simulink model "c09f12_01_avn"  (R2012b)
settings: Solver=ode45  StartTime=0.0  StopTime="(2^(7+2))  * (2^8)"  RelTol=1e-3
undefined symbols (not defined in the file): Down, pfb_coeff_gen_calc, Up, xlipgetpartsetting
libraries: xbsIndex_r4 x7041, casper_library_misc x193, xps_library x58, casper_library_delays x50, simulink x16, dspsigops x12, casper_library_flow_control x5, xbsReplacements_r4 x4, casper_library_ffts_twiddle x2, casper_library_multipliers x2, casper_library_reorder x1
(part 3 of 77)

== system c09f12_01_avn/calc_adc_sum_sq ==
  In1 : Inport
  In2 : Inport  Port=2
  In3 : Inport  Port=3
  In4 : Inport  Port=4
  Accumulator : xbsIndex_r4/Accumulator  operation=Add  n_bits=32  overflow=Wrap  scale=1  rst=on  infoeditControl=reset for floating point data type must be asserted for a minimum of 2 cycles  hasbypass=off  en=off  latency=0  dbl_ovrd=off  msb_inp=100  msb=100  lsb=-100  use_behavioral_HDL=off  implementation=DSP48  block_type=accum
      settings: xl_area=[0, 0, 0, 0, 0, 0, 0]  block_version=10.1.3
  Convert1 : xbsIndex_r4/Convert  gui_display_data_type=Fixed-point  arith_type=Unsigned  n_bits=32  bin_pt=0  float_type=Single  exp_bits=8  fraction_bits=24  quantization=Truncate  overflow=Wrap  en=off  latency=0  dbl_ovrd=off  pipeline=off  block_type=convert
      settings: block_version=11.4
  Counter : xbsIndex_r4/Counter  cnt_type=Free Running  cnt_to=Inf  operation=Up  start_count=0  cnt_by_val=1  arith_type=Unsigned  n_bits=2  bin_pt=0  load_pin=off  rst=off  en=off  explicit_period=off  period=1  dbl_ovrd=off  use_behavioral_HDL=off  implementation=Fabric  use_rpm=on  block_type=counter
      settings: xl_area=[0, 0, 0, 0, 0, 0, 0]
  Counter1 : xbsIndex_r4/Counter  cnt_type=Free Running  cnt_to=Inf  operation=Up  start_count=0  cnt_by_val=1  arith_type=Unsigned  n_bits=16  bin_pt=0  load_pin=off  rst=off  en=off  explicit_period=on  period=1  dbl_ovrd=off  use_behavioral_HDL=off  implementation=DSP48  use_rpm=on  block_type=counter
      settings: xl_area=[0, 0, 0, 0, 0, 0, 0]
  Delay : xbsIndex_r4/Delay  rst=off  infoeditControl=Selection of Reset will increase slice count due to use of real FFs and instead of SRLs  en=off  latency=1  dbl_ovrd=off  reg_retiming=on  block_type=delay
      settings: block_version=11.4
  Delay1 : xbsIndex_r4/Delay  rst=off  infoeditControl=Selection of Reset will increase slice count due to use of real FFs and instead of SRLs  en=off  latency=1  dbl_ovrd=off  reg_retiming=on  block_type=delay
      settings: block_version=11.4
  Mult : xbsIndex_r4/Mult  precision=Full  arith_type="Signed  (2's comp)"  n_bits=8  bin_pt=2  quantization=Truncate  overflow=Wrap  en=off  latency=2  dbl_ovrd=off  use_behavioral_HDL=on  opt=Speed  use_embedded=on  optimum_pipeline=off  pipeline=on  use_rpm=on  placement_style=Rectangular shape  block_type=mult
      settings: xl_area=[0, 0, 0, 0, 0, 0, 0]  block_version=10.1.3
  Mux : xbsIndex_r4/Mux  inputs=4  en=off  latency=1  precision=Full  arith_type="Signed  (2's comp)"  n_bits=8  bin_pt=2  quantization=Truncate  overflow=Wrap  dbl_ovrd=off  block_type=mux
      settings: xl_area=[0, 0, 0, 0, 0, 0, 0]
  Register : xbsIndex_r4/Register  init=0  rst=off  en=on  dbl_ovrd=off  block_type=register
      settings: xl_area=[0, 0, 0, 0, 0, 0, 0]
  Slice : xbsIndex_r4/Slice  nbits=1  boolean_output=on  mode=Upper Bit Location + Width  bit1=0  base1=MSB of Input  bit0=0  base0=LSB of Input  dbl_ovrd=off  block_type=slice
      settings: block_version=10.1.3
  edge_detect1 : Subsystem  AncestorBlock=casper_library_misc/edge_detect  mask(edge_detect){edge=Falling, polarity=Active High, x_in=[0 0.08 0.08 0.16 0.16 0.24 0.24 0.32 0.32 0.4], y_in=[1  1 -1 -1 -1 -1 -1 -1 -1 -1], x_out=[0.6 0.68 0.68 0.76 0.76 0.84 0.84 0.92 0.92 1], y_out=[-1 -1  1  1 -1 -1 -1 -1 -1 -1]}
      mask prompts: edge "Edge Type"; polarity "Output Polarity"; x_in "Input X Positions"; y_in "Input Y Positions"; x_out "Output X Positions"; y_out "Output Y Positions"
      mask help: Output is active for one-cycle after each edge of the specified type (i.e. rising, falling or both).
      mask init: same as c09f12_01_avn/edge_detect2
      settings: AttributesFormatString=|
      | falling edges
      | active high
      mask Help: Output is active for one-cycle after each edge of the specified type (i.e. rising, falling, or both).  Latency is zero.
      mask TypeOptions edge: Rising | Falling | Both
      mask TypeOptions polarity: Active High | Active Low
      mask Display:
      | plot(x_in_num,0.5+y_in_num*0.2);
      | plot(x_out_num,0.5+y_out_num*0.2);
  sum_sq : Outport
  wires:
  Mult/1 -> Delay/1
  Accumulator/1 -> Register/1
  Register/1 -> Convert1/1
  Mux/1 -> Mult/1, Mult/2
  Counter/1 -> Mux/1
  Counter1/1 -> Slice/1
  Slice/1 -> edge_detect1/1(in)
  edge_detect1/1(out) -> Delay1/1
  In1/1 -> Mux/2
  In3/1 -> Mux/3
  In2/1 -> Mux/4
  In4/1 -> Mux/5
  Convert1/1 -> sum_sq/1
  Delay/1 -> Accumulator/1
  Delay1/1 -> Accumulator/2, Register/2

== system c09f12_01_avn/calc_adc_sum_sq1 ==
  In1 : Inport
  In2 : Inport  Port=2
  In3 : Inport  Port=3
  In4 : Inport  Port=4
  Accumulator : xbsIndex_r4/Accumulator  operation=Add  n_bits=32  overflow=Wrap  scale=1  rst=on  infoeditControl=reset for floating point data type must be asserted for a minimum of 2 cycles  hasbypass=off  en=off  latency=0  dbl_ovrd=off  msb_inp=100  msb=100  lsb=-100  use_behavioral_HDL=off  implementation=DSP48  block_type=accum
      settings: xl_area=[0, 0, 0, 0, 0, 0, 0]  block_version=10.1.3
  Convert1 : xbsIndex_r4/Convert  gui_display_data_type=Fixed-point  arith_type=Unsigned  n_bits=32  bin_pt=0  float_type=Single  exp_bits=8  fraction_bits=24  quantization=Truncate  overflow=Wrap  en=off  latency=0  dbl_ovrd=off  pipeline=off  block_type=convert
      settings: block_version=11.4
  Counter : xbsIndex_r4/Counter  cnt_type=Free Running  cnt_to=Inf  operation=Up  start_count=0  cnt_by_val=1  arith_type=Unsigned  n_bits=2  bin_pt=0  load_pin=off  rst=off  en=off  explicit_period=off  period=1  dbl_ovrd=off  use_behavioral_HDL=off  implementation=Fabric  use_rpm=on  block_type=counter
      settings: xl_area=[0, 0, 0, 0, 0, 0, 0]
  Counter1 : xbsIndex_r4/Counter  cnt_type=Free Running  cnt_to=Inf  operation=Up  start_count=0  cnt_by_val=1  arith_type=Unsigned  n_bits=16  bin_pt=0  load_pin=off  rst=off  en=off  explicit_period=on  period=1  dbl_ovrd=off  use_behavioral_HDL=off  implementation=DSP48  use_rpm=on  block_type=counter
      settings: xl_area=[0, 0, 0, 0, 0, 0, 0]
  Delay : xbsIndex_r4/Delay  rst=off  infoeditControl=Selection of Reset will increase slice count due to use of real FFs and instead of SRLs  en=off  latency=1  dbl_ovrd=off  reg_retiming=on  block_type=delay
      settings: block_version=11.4
  Delay1 : xbsIndex_r4/Delay  rst=off  infoeditControl=Selection of Reset will increase slice count due to use of real FFs and instead of SRLs  en=off  latency=1  dbl_ovrd=off  reg_retiming=on  block_type=delay
      settings: block_version=11.4
  Mult : xbsIndex_r4/Mult  precision=Full  arith_type="Signed  (2's comp)"  n_bits=8  bin_pt=2  quantization=Truncate  overflow=Wrap  en=off  latency=2  dbl_ovrd=off  use_behavioral_HDL=on  opt=Speed  use_embedded=on  optimum_pipeline=off  pipeline=on  use_rpm=on  placement_style=Rectangular shape  block_type=mult
      settings: xl_area=[0, 0, 0, 0, 0, 0, 0]  block_version=10.1.3
  Mux : xbsIndex_r4/Mux  inputs=4  en=off  latency=1  precision=Full  arith_type="Signed  (2's comp)"  n_bits=8  bin_pt=2  quantization=Truncate  overflow=Wrap  dbl_ovrd=off  block_type=mux
      settings: xl_area=[0, 0, 0, 0, 0, 0, 0]
  Register : xbsIndex_r4/Register  init=0  rst=off  en=on  dbl_ovrd=off  block_type=register
      settings: xl_area=[0, 0, 0, 0, 0, 0, 0]
  Slice : xbsIndex_r4/Slice  nbits=1  boolean_output=on  mode=Upper Bit Location + Width  bit1=0  base1=MSB of Input  bit0=0  base0=LSB of Input  dbl_ovrd=off  block_type=slice
      settings: block_version=10.1.3
  edge_detect1 : Subsystem  AncestorBlock=casper_library_misc/edge_detect  mask(edge_detect){edge=Falling, polarity=Active High, x_in=[0 0.08 0.08 0.16 0.16 0.24 0.24 0.32 0.32 0.4], y_in=[1  1 -1 -1 -1 -1 -1 -1 -1 -1], x_out=[0.6 0.68 0.68 0.76 0.76 0.84 0.84 0.92 0.92 1], y_out=[-1 -1  1  1 -1 -1 -1 -1 -1 -1]}
      mask prompts: edge "Edge Type"; polarity "Output Polarity"; x_in "Input X Positions"; y_in "Input Y Positions"; x_out "Output X Positions"; y_out "Output Y Positions"
      mask help: Output is active for one-cycle after each edge of the specified type (i.e. rising, falling or both).
      mask init: same as c09f12_01_avn/edge_detect2
      settings: AttributesFormatString=|
      | falling edges
      | active high
      mask Help: Output is active for one-cycle after each edge of the specified type (i.e. rising, falling, or both).  Latency is zero.
      mask TypeOptions edge: Rising | Falling | Both
      mask TypeOptions polarity: Active High | Active Low
      mask Display:
      | plot(x_in_num,0.5+y_in_num*0.2);
      | plot(x_out_num,0.5+y_out_num*0.2);
  sum_sq : Outport
  wires:
  Delay1/1 -> Register/2, Accumulator/2
  Delay/1 -> Accumulator/1
  Convert1/1 -> sum_sq/1
  In4/1 -> Mux/5
  In2/1 -> Mux/4
  In3/1 -> Mux/3
  In1/1 -> Mux/2
  edge_detect1/1(out) -> Delay1/1
  Slice/1 -> edge_detect1/1(in)
  Counter1/1 -> Slice/1
  Counter/1 -> Mux/1
  Mux/1 -> Mult/2, Mult/1
  Register/1 -> Convert1/1
  Accumulator/1 -> Register/1
  Mult/1 -> Delay/1

== system c09f12_01_avn/cd_local_time ==
  note: A reset pulse resets
      | the clock which starts
      | counting at the next sync
  reset : Inport
  sync : Inport  Port=2
  Delay : xbsIndex_r4/Delay  rst=off  infoeditControl=Selection of Reset will increase slice count due to use of real FFs and instead of SRLs  en=off  latency=1  dbl_ovrd=off  reg_retiming=on  block_type=delay
  Register : xbsIndex_r4/Register  init=0  rst=on  en=on  dbl_ovrd=off  block_type=register
  clock : xbsIndex_r4/Counter  cnt_type=Free Running  cnt_to=Inf  operation=Up  start_count=0  cnt_by_val=1  arith_type=Unsigned  n_bits=64  bin_pt=0  load_pin=off  rst=on  en=on  explicit_period=on  period=1  dbl_ovrd=off  use_behavioral_HDL=off  implementation=Fabric  use_rpm=on  block_type=counter
  edge_detect1 : casper_library_misc/edge_detect  edge=Rising  polarity=Active High  x_in=[0 0.08 0.08 0.16 0.16 0.24 0.24 0.32 0.32 0.4]  y_in="[-1 -1  1  1  1  1  1  1  1  1]"  x_out=[0.6 0.68 0.68 0.76 0.76 0.84 0.84 0.92 0.92 1]  y_out="[-1 -1  1  1 -1 -1 -1 -1 -1 -1]"
  time : Outport
  wires:
  clock/1 -> time/1
  sync/1 -> Register/1, Register/3
  reset/1 -> Register/2, edge_detect1/1
  Register/1 -> clock/2
  edge_detect1/1 -> Delay/1
  Delay/1 -> clock/1

== system c09f12_01_avn/coarse ==
  sync : Inport
  data0 : Inport  Port=2
  data1 : Inport  Port=3
  fft_shift : Inport  Port=4
  channel_select : Inport  Port=5
  debug_polsel : Inport  Port=6
  debug_chansel : Inport  Port=7
  debug_chan : Inport  Port=8
  1st_shift : Subsystem  mask{shift=fftShift, latency=0}
      mask prompts: shift "Number bits to shift right by"; latency "Shift latency"
  1st_shift1 : Subsystem  mask{shift=fftShift, latency=0}
      mask prompts: shift "Number bits to shift right by"; latency "Shift latency"
  Delay1 : xbsIndex_r4/Delay  rst=off  infoeditControl=Selection of Reset will increase slice count due to use of real FFs and instead of SRLs  en=off  latency=1  dbl_ovrd=off  reg_retiming=on  block_type=delay
      settings: block_version=11.4
  Delay2 : xbsIndex_r4/Delay  rst=off  infoeditControl=Selection of Reset will increase slice count due to use of real FFs and instead of SRLs  en=off  latency=1  dbl_ovrd=off  reg_retiming=on  block_type=delay
      settings: block_version=11.4
  Delay3 : xbsIndex_r4/Delay  rst=off  infoeditControl=Selection of Reset will increase slice count due to use of real FFs and instead of SRLs  en=off  latency=1  dbl_ovrd=off  reg_retiming=on  block_type=delay
      settings: block_version=11.4
  Mux1 : xbsIndex_r4/Mux  inputs=2  en=off  latency=1  precision=Full  arith_type=Unsigned  n_bits=16  bin_pt=14  quantization=Truncate  overflow=Wrap  dbl_ovrd=off  block_type=mux
      settings: block_version=11.4
  Mux2 : xbsIndex_r4/Mux  inputs=2  en=off  latency=1  precision=Full  arith_type=Unsigned  n_bits=16  bin_pt=14  quantization=Truncate  overflow=Wrap  dbl_ovrd=off  block_type=mux
      settings: block_version=11.4
  Slice3 : xbsIndex_r4/Slice  nbits=1  boolean_output=off  mode=Lower Bit Location + Width  bit1=0  base1=MSB of Input  bit0=0  base0=LSB of Input  dbl_ovrd=off  block_type=slice
      settings: block_version=10.1.3
  Terminator7 : Terminator
  bus_create1 : Subsystem  AncestorBlock=casper_library_flow_control/bus_create  mask(bus_create){inputNum=2}
      mask prompts: inputNum "Number of inputs:"
      mask init:
      | bus_create_init(gcb,...
      |     'inputNum', inputNum);
  bus_create2 : casper_library_flow_control/bus_create  inputNum=2
  bus_create4 : Subsystem  AncestorBlock=casper_library_flow_control/bus_create  mask(bus_create){inputNum=2}
      mask prompts: inputNum "Number of inputs:"
      mask init:
      | bus_create_init(gcb,...
      |     'inputNum', inputNum);
  bus_expand1 : Subsystem  AncestorBlock=casper_library_flow_control/bus_expand  mask(bus_expand){mode=divisions of equal size, outputNum=4, outputWidth=8, outputBinaryPt=0, outputArithmeticType=0, show_format=on, outputToWorkspace=off, variablePrefix=adc0_d, outputToModelAsWell=on}
      mask prompts: outputNum "Number of outputs:"; outputWidth "Output width:"; outputBinaryPt "Output binary point position:"; outputArithmeticType "Output arithmetic type: (Unsigned=0, Signed=1, Boolean=2)"; show_format "Print format string?"; outputToWorkspace "Output to workspace?"; variablePrefix "Variable name prefix:"; outputToModelAsWell "Output to model as well?"
      mask help:
      | Expands a 'bus' made using a bus_create or Xilinx
      | concat block.
      | The input will be divided into the specified number
      | of outputs with the specified arithmetic types.
      | Divisions are made from most significant bit.
      mask init: same as c09f12_01_avn/bus_expand6
      settings: AttributesFormatString=4 outputs: uf8.0,uf8.0,uf8.0,uf8.0,
      mask TypeOptions mode: divisions of equal size | divisions of arbitrary size
      mask Callback mode: bus_expand_callback();
      mask Callback outputWidth: bus_expand_callback();
      mask Callback outputToWorkspace: bus_expand_callback();
  bus_expand2 : Subsystem  AncestorBlock=casper_library_flow_control/bus_expand  mask(bus_expand){mode=divisions of equal size, outputNum=4, outputWidth=8, outputBinaryPt=0, outputArithmeticType=0, show_format=on, outputToWorkspace=off, variablePrefix=adc0_d, outputToModelAsWell=on}
      mask prompts: outputNum "Number of outputs:"; outputWidth "Output width:"; outputBinaryPt "Output binary point position:"; outputArithmeticType "Output arithmetic type: (Unsigned=0, Signed=1, Boolean=2)"; show_format "Print format string?"; outputToWorkspace "Output to workspace?"; variablePrefix "Variable name prefix:"; outputToModelAsWell "Output to model as well?"
      mask help:
      | Expands a 'bus' made using a bus_create or Xilinx
      | concat block.
      | The input will be divided into the specified number
      | of outputs with the specified arithmetic types.
      | Divisions are made from most significant bit.
      mask init: same as c09f12_01_avn/bus_expand6
      settings: AttributesFormatString=4 outputs: uf8.0,uf8.0,uf8.0,uf8.0,
      mask TypeOptions mode: divisions of equal size | divisions of arbitrary size
      mask Callback mode: bus_expand_callback();
      mask Callback outputWidth: bus_expand_callback();
      mask Callback outputToWorkspace: bus_expand_callback();
  crs_snap : Subsystem
  fft_wideband_real0 : Subsystem  AncestorBlock=casper_library_ffts/fft_wideband_real  mask(fft_wideband_real){FFTSize=9, n_inputs=2, input_bit_width=18, coeff_bit_width=18, unscramble=on, add_latency=2, mult_latency=3, bram_latency=3, conv_latency=2, input_latency=1, biplex_direct_latency=1, quantization=Round  (unbiased: Even Values), overflow=Wrap, arch=Virtex5, opt_target=logic, coeffs_bit_limit=8, delays_bit_limit=8, mult_spec=2, hardcode_shifts=off, shift_schedule=, dsp48_adders=on}
      mask prompts: FFTSize "Size of FFT: (2^? pts)"; n_inputs "Number of Simultaneous Inputs: (2^?)"; input_bit_width "Input/Output Bit Width"; coeff_bit_width "Coefficient Bit Width"; unscramble "Unscramble output (ie, put channels in canonical order)"; add_latency "Add Latency"; mult_latency "Mult Latency"; bram_latency "BRAM Latency"; conv_latency "Convert Latency"; input_latency "Input Latency"; biplex_direct_latency "Latency between biplexes and fft_direct"; quantization "Quantization Behavior"; overflow "Overflow Behavior"; arch "Architecture"; opt_target "Use less"; coeffs_bit_limit "Number bits above which to store stage's coefficients in BRAM (2^? bits)"; delays_bit_limit "Number bits above which to store stage's delays in BRAM (2^? bits)"; mult_spec "Multiplier impl. (0=core, 1=embedded, 2=behavioural) (left=1st stage, or just one value)"; hardcode_shifts "Hardcode shift schedule"; shift_schedule "Shift schedule"; dsp48_adders "DSP48 adders in butterfly"
      mask help: A real-sampled wideband FFT.
      mask init:
      | fft_wideband_real_init(gcb, ...
      |     'FFTSize', FFTSize, ...
      |     'n_inputs', n_inputs, ...
      |     'input_bit_width', input_bit_width, ...
      |     'coeff_bit_width', coeff_bit_width, ...
      |     'unscramble', unscramble, ...
      |     'add_latency', add_latency, ...
      |     'mult_latency', mult_latency, ...
      |     'bram_latency', bram_latency, ...
      |     'conv_latency', conv_latency, ...
      |     'input_latency', input_latency, ...
      |     'biplex_direct_latency', biplex_direct_latency, ...
      |     'quantization', quantization, ...
      |     'overflow', overflow, ...
      |     'arch', arch, ...
      |     'opt_target', opt_target, ...
      |     'coeffs_bit_limit', coeffs_bit_limit, ...
      |     'delays_bit_limit', delays_bit_limit, ...
      |     'mult_spec', mult_spec, ...
      |     'hardcode_shifts', hardcode_shifts, ...
      |     'shift_schedule', shift_schedule, ...
      |     'dsp48_adders', dsp48_adders);
      settings: CopyFcn=fft_wideband_real_init(gcb);
      settings: AttributesFormatString=|
      | 9 stages
      | (18,18)
      | Round  (unbiased: Even Values)
      | Wrap
      mask Help: eval('xlWeb(''http://casper.berkeley.edu/wiki/Fft_wideband_real'')')
      mask TypeOptions quantization: Truncate | Round  (unbiased: +/- Inf) | Round  (unbiased: Even Values)
      mask TypeOptions overflow: Wrap | Saturate | Error
      mask TypeOptions arch: Virtex2Pro | Virtex5
      mask Callback arch: fft_callback_arch(gcb);
      mask TypeOptions opt_target: logic | multipliers
      mask Callback hardcode_shifts:
      | hardcode_shifts = get_param(gcb, 'hardcode_shifts');
      | set_param_state(gcb, 'shift_schedule', hardcode_shifts);
      mask Callback dsp48_adders: fft_callback_dsp48_adders(gcb);
  fft_wideband_real1 : Subsystem  AncestorBlock=casper_library_ffts/fft_wideband_real  mask(fft_wideband_real){FFTSize=9, n_inputs=2, input_bit_width=18, coeff_bit_width=18, unscramble=on, add_latency=2, mult_latency=3, bram_latency=3, conv_latency=2, input_latency=1, biplex_direct_latency=1, quantization=Round  (unbiased: Even Values), overflow=Wrap, arch=Virtex5, opt_target=logic, coeffs_bit_limit=8, delays_bit_limit=8, mult_spec=2, hardcode_shifts=off, shift_schedule=, dsp48_adders=on}
      mask prompts: FFTSize "Size of FFT: (2^? pts)"; n_inputs "Number of Simultaneous Inputs: (2^?)"; input_bit_width "Input/Output Bit Width"; coeff_bit_width "Coefficient Bit Width"; unscramble "Unscramble output (ie, put channels in canonical order)"; add_latency "Add Latency"; mult_latency "Mult Latency"; bram_latency "BRAM Latency"; conv_latency "Convert Latency"; input_latency "Input Latency"; biplex_direct_latency "Latency between biplexes and fft_direct"; quantization "Quantization Behavior"; overflow "Overflow Behavior"; arch "Architecture"; opt_target "Use less"; coeffs_bit_limit "Number bits above which to store stage's coefficients in BRAM (2^? bits)"; delays_bit_limit "Number bits above which to store stage's delays in BRAM (2^? bits)"; mult_spec "Multiplier impl. (0=core, 1=embedded, 2=behavioural) (left=1st stage, or just one value)"; hardcode_shifts "Hardcode shift schedule"; shift_schedule "Shift schedule"; dsp48_adders "DSP48 adders in butterfly"
      mask help: A real-sampled wideband FFT.
      mask init: same as c09f12_01_avn/coarse/fft_wideband_real0
      settings: CopyFcn=fft_wideband_real_init(gcb);
      settings: AttributesFormatString=|
      | 9 stages
      | (18,18)
      | Round  (unbiased: Even Values)
      | Wrap
      mask Help: eval('xlWeb(''http://casper.berkeley.edu/wiki/Fft_wideband_real'')')
      mask TypeOptions quantization: Truncate | Round  (unbiased: +/- Inf) | Round  (unbiased: Even Values)
      mask TypeOptions overflow: Wrap | Saturate | Error
      mask TypeOptions arch: Virtex2Pro | Virtex5
      mask Callback arch: fft_callback_arch(gcb);
      mask TypeOptions opt_target: logic | multipliers
      mask Callback hardcode_shifts:
      | hardcode_shifts = get_param(gcb, 'hardcode_shifts');
      | set_param_state(gcb, 'shift_schedule', hardcode_shifts);
      mask Callback dsp48_adders: fft_callback_dsp48_adders(gcb);
  pfb_fir_real : Subsystem  AncestorBlock=casper_library_pfbs/pfb_fir_real  mask(pfb_fir_real){PFBSize=5, TotalTaps=2, WindowType=hamming, n_inputs=2, MakeBiplex=on, BitWidthIn=8, BitWidthOut=18, CoeffBitWidth=18, CoeffDistMem=off, add_latency=2, mult_latency=3, bram_latency=3, fan_latency=1, conv_latency=1, quantization=Round  (unbiased: Even Values), fwidth=1, mult_spec=2, adder_folding=on, adder_imp=Fabric, coeffs_share=off}
      mask prompts: PFBSize "Size of PFB: (2^? pnts)"; TotalTaps "Total Number of Taps:"; WindowType "Windowing Function:"; n_inputs "Number of Simultaneous Inputs: (2^?)"; MakeBiplex "Make Biplex?"; BitWidthIn "Input Bitwidth:"; BitWidthOut "Output Bitwidth:"; CoeffBitWidth "Coefficient Bitwidth:"; CoeffDistMem "Use Distributed Memory for Coeffs"; add_latency "Add Latency"; mult_latency "Mult Latency"; bram_latency "BRAM Latency"; fan_latency "Fanout latency"; conv_latency "Convert latency"; quantization "Quantization Behavior"; fwidth "Bin Width Scaling (normal=1)"; mult_spec "Multiplier specification (0=core, 1=embedded, 2=behavioural) (left=1st tap, or just one value)"; adder_folding "Fold adders into DSPs"; adder_imp "Adder implementation"; coeffs_share "Share coefficients between polarisations (use less BRAM)?"
      mask help:
      | Fold adders into DSPs: Causes adders to be absorbed into DSP blocks (supported in Virtex5)
      | Adder implementation: Cores using Fabric or DSP48 or behavioral HDL
      mask init:
      | pfb_fir_real_init(gcb, ...
      |     'PFBSize', PFBSize, ...
      |     'TotalTaps', TotalTaps, ...
      |     'WindowType', WindowType, ...
      |     'n_inputs', n_inputs, ...
      |     'MakeBiplex', MakeBiplex, ...
      |     'BitWidthIn', BitWidthIn, ...
      |     'BitWidthOut', BitWidthOut, ...
      |     'CoeffBitWidth', CoeffBitWidth, ...
      |     'CoeffDistMem', CoeffDistMem, ...
      |     'add_latency', add_latency, ...
      |     'mult_latency', mult_latency, ...
      |     'bram_latency', bram_latency, ...
      |     'fan_latency', fan_latency, ...
      |     'conv_latency', conv_latency, ...
      |     'quantization', quantization, ...
      |     'fwidth', fwidth, ...
      |     'mult_spec', mult_spec, ...
      |     'adder_folding', adder_folding, ...
      |     'adder_imp', adder_imp, ...
      |     'coeffs_share', coeffs_share);
      settings: AttributesFormatString=taps=2, add_latency=2
      mask Help: eval('xlWeb(''http://casper.berkeley.edu/wiki/Pfb_fir_real'')')
      mask Callback TotalTaps:
      | %num_taps = eval(get_param(gcb, 'TotalTaps'));
      | %old_vec = eval(get_param(gcb, 'mult_spec'));=-0l
      | 
      | %vec = 2.*ones(1,num_taps);
      | %old_size = length(old_vec);
      | 
      | %if(old_size <= num_taps),
      | %    new_size = old_size;
      | %else,
      | %    new_size = num_taps;
      | %end
      | 
      | %for n = 1:new_size, vec(n) = old_vec(n); end
      | %set_param(gcb, 'mult_spec', mat2str(vec));
      mask TypeOptions WindowType: bartlett | barthannwin | blackman | blackmanharris | bohamwin | chebwin | flattopwin | gausswin | hamming | hann | kaiser | nuttallwin | parzenwin | rectwin | tukeywin | triang | userwindow
      mask TypeOptions quantization: Truncate | Round  (unbiased: +/- Inf) | Round  (unbiased: Even Values)
      mask TypeOptions adder_imp: Behavioral | Fabric | DSP48
  sync_out : Outport
  data_out : Outport  Port=2
  fft_of0 : Outport  Port=3
  fft_of1 : Outport  Port=4
  snap72 : Outport  Port=5
  wires:
  1st_shift/1(sync_out) -> fft_wideband_real0/1(sync)
  fft_shift/1 -> fft_wideband_real0/2(shift), fft_wideband_real1/2(shift)
  1st_shift/2(dout1) -> fft_wideband_real0/3(in0)
  1st_shift/3(dout2) -> fft_wideband_real0/4(in1)
  1st_shift/4(dout3) -> fft_wideband_real0/5(in2)
  1st_shift/5(dout4) -> fft_wideband_real0/6(in3)
  channel_select/1 -> Slice3/1
  Slice3/1 -> Mux1/1, Mux2/1
  Delay1/1 -> sync_out/1
  Delay2/1 -> fft_of0/1
  bus_create4/1(bus_out) -> crs_snap/3(data_pol0)
  fft_wideband_real0/1(sync_out) -> Delay1/1, crs_snap/2(sync)
  fft_wideband_real0/4(of) -> Delay2/1
  fft_wideband_real0/2(out0) -> Mux1/2, bus_create4/1(in1)
  fft_wideband_real0/3(out1) -> Mux1/3, bus_create4/2(in2)
  pfb_fir_real/1(sync_out) -> 1st_shift/1(sync_in), 1st_shift1/1(sync_in)
  pfb_fir_real/2(pol1_out1) -> 1st_shift/2(din1)
  pfb_fir_real/3(pol1_out2) -> 1st_shift/3(din2)
  pfb_fir_real/4(pol1_out3) -> 1st_shift/4(din3)
  pfb_fir_real/5(pol1_out4) -> 1st_shift/5(din4)
  1st_shift1/1(sync_out) -> fft_wideband_real1/1(sync)
  1st_shift1/2(dout1) -> fft_wideband_real1/3(in0)
  1st_shift1/3(dout2) -> fft_wideband_real1/4(in1)
  1st_shift1/4(dout3) -> fft_wideband_real1/5(in2)
  1st_shift1/5(dout4) -> fft_wideband_real1/6(in3)
  bus_create1/1(bus_out) -> crs_snap/4(data_pol1)
  fft_wideband_real1/4(of) -> Delay3/1
  fft_wideband_real1/2(out0) -> bus_create1/1(in1), Mux2/2
  fft_wideband_real1/3(out1) -> bus_create1/2(in2), Mux2/3
  Delay3/1 -> fft_of1/1
  pfb_fir_real/6(pol2_out1) -> 1st_shift1/2(din1)
  pfb_fir_real/7(pol2_out2) -> 1st_shift1/3(din2)
  pfb_fir_real/8(pol2_out3) -> 1st_shift1/4(din3)
  pfb_fir_real/9(pol2_out4) -> 1st_shift1/5(din4)
  fft_wideband_real1/1(sync_out) -> Terminator7/1
  Mux2/1 -> bus_create2/2
  bus_create2/1 -> data_out/1
  Mux1/1 -> bus_create2/1
  sync/1 -> pfb_fir_real/1(sync)
  data0/1 -> bus_expand2/1(bus_in)
  data1/1 -> bus_expand1/1(bus_in)
  debug_polsel/1 -> crs_snap/1(pol_select)
  crs_snap/1(coarse_debug) -> snap72/1
  bus_expand2/1(msb_out4) -> pfb_fir_real/2(pol1_in1)
  bus_expand2/2(out3) -> pfb_fir_real/3(pol1_in2)
  bus_expand2/3(out2) -> pfb_fir_real/4(pol1_in3)
  bus_expand2/4(lsb_out1) -> pfb_fir_real/5(pol1_in4)
  bus_expand1/1(msb_out4) -> pfb_fir_real/6(pol2_in1)
  bus_expand1/2(out3) -> pfb_fir_real/7(pol2_in2)
  bus_expand1/3(out2) -> pfb_fir_real/8(pol2_in3)
  bus_expand1/4(lsb_out1) -> pfb_fir_real/9(pol2_in4)
  debug_chansel/1 -> crs_snap/5(select_chan)
  debug_chan/1 -> crs_snap/6(selected_chan)

== system c09f12_01_avn/coarse_delay ==
  mrst : Inport
  sync : Inport  Port=2
  cd_lt : Inport  Port=3
  load_now : Inport  Port=4
  data0 : Inport  Port=5
  arm0 : Inport  Port=6
  ld_time0 : Inport  Port=7
  ld_val0 : Inport  Port=8
  data1 : Inport  Port=9
  arm1 : Inport  Port=10
  ld_time1 : Inport  Port=11
  ld_val1 : Inport  Port=12
  Concat1 : xbsIndex_r4/Concat  num_inputs=2  dbl_ovrd=off  block_type=concat
  Concat4 : xbsIndex_r4/Concat  num_inputs=2  dbl_ovrd=off  block_type=concat
  Constant1 : xbsIndex_r4/Constant  const=0  gui_display_data_type=Fixed-point  arith_type=Boolean  n_bits=1  bin_pt=0  preci_type=Single  exp_width=8  frac_width=24  explicit_period=on  period=1  equ=P=C  opselect=C  inp2=PCIN>>17  opr=+  inp1=P  carry=CIN  dbl_ovrd=off  block_type=constant
      settings: block_version=11.4
  Constant19 : xbsIndex_r4/Constant  const=0  gui_display_data_type=Fixed-point  arith_type=Boolean  n_bits=1  bin_pt=0  preci_type=Single  exp_width=8  frac_width=24  explicit_period=on  period=1  equ=P=C  opselect=C  inp2=PCIN>>17  opr=+  inp1=P  carry=CIN  dbl_ovrd=off  block_type=constant
      settings: block_version=11.4
  Logical1 : xbsIndex_r4/Logical  logical_function=OR  inputs=2  en=off  latency=0  precision=Full  arith_type=Unsigned  n_bits=16  bin_pt=0  align_bp=on  dbl_ovrd=off  block_type=logical
      settings: block_version=11.4
  Logical12 : xbsIndex_r4/Logical  logical_function=OR  inputs=2  en=off  latency=0  precision=Full  arith_type=Unsigned  n_bits=16  bin_pt=0  align_bp=on  dbl_ovrd=off  block_type=logical
      settings: block_version=11.4
  Slice1 : xbsIndex_r4/Slice  nbits=16  boolean_output=off  mode=Lower Bit Location + Width  bit1=0  base1=MSB of Input  bit0=0*16  base0=LSB of Input  dbl_ovrd=off  block_type=slice
      settings: block_version=10.1.3
  Slice15 : xbsIndex_r4/Slice  nbits=16  boolean_output=off  mode=Lower Bit Location + Width  bit1=0  base1=MSB of Input  bit0=0*16  base0=LSB of Input  dbl_ovrd=off  block_type=slice
      settings: block_version=10.1.3
  Slice16 : xbsIndex_r4/Slice  nbits=16  boolean_output=off  mode=Lower Bit Location + Width  bit1=0  base1=MSB of Input  bit0=16*3+15  base0=LSB of Input  dbl_ovrd=off  block_type=slice
      settings: block_version=10.1.3
  Slice17 : xbsIndex_r4/Slice  nbits=16  boolean_output=off  mode=Lower Bit Location + Width  bit1=0  base1=MSB of Input  bit0=16*1  base0=LSB of Input  dbl_ovrd=off  block_type=slice
      settings: block_version=10.1.3
  Slice18 : xbsIndex_r4/Slice  nbits=15  boolean_output=off  mode=Lower Bit Location + Width  bit1=0  base1=MSB of Input  bit0=16*2  base0=LSB of Input  dbl_ovrd=off  block_type=slice
      settings: block_version=10.1.3
  Slice19 : xbsIndex_r4/Slice  nbits=16  boolean_output=off  mode=Lower Bit Location + Width  bit1=0  base1=MSB of Input  bit0=16*2+15  base0=LSB of Input  dbl_ovrd=off  block_type=slice
      settings: block_version=10.1.3
  Slice2 : xbsIndex_r4/Slice  nbits=16  boolean_output=off  mode=Lower Bit Location + Width  bit1=0  base1=MSB of Input  bit0=16*3+15  base0=LSB of Input  dbl_ovrd=off  block_type=slice
      settings: block_version=10.1.3
  Slice3 : xbsIndex_r4/Slice  nbits=16  boolean_output=off  mode=Lower Bit Location + Width  bit1=0  base1=MSB of Input  bit0=16*1  base0=LSB of Input  dbl_ovrd=off  block_type=slice
      settings: block_version=10.1.3
  Slice4 : xbsIndex_r4/Slice  nbits=15  boolean_output=off  mode=Lower Bit Location + Width  bit1=0  base1=MSB of Input  bit0=16*2  base0=LSB of Input  dbl_ovrd=off  block_type=slice
      settings: block_version=10.1.3
  Slice5 : xbsIndex_r4/Slice  nbits=16  boolean_output=off  mode=Lower Bit Location + Width  bit1=0  base1=MSB of Input  bit0=16*2+15  base0=LSB of Input  dbl_ovrd=off  block_type=slice
      settings: block_version=10.1.3
  Terminator{1..11,14..15} (13 alike) : Terminator
  bus_create1 : Subsystem  AncestorBlock=casper_library_flow_control/bus_create  mask(bus_create){inputNum=2}
      mask prompts: inputNum "Number of inputs:"
      mask init:
      | bus_create_init(gcb,...
      |     'inputNum', inputNum);
  bus_create2 : Subsystem  AncestorBlock=casper_library_flow_control/bus_create  mask(bus_create){inputNum=4}
      mask prompts: inputNum "Number of inputs:"
      mask init:
      | bus_create_init(gcb,...
      |     'inputNum', inputNum);
  bus_create4 : Subsystem  AncestorBlock=casper_library_flow_control/bus_create  mask(bus_create){inputNum=4}
      mask prompts: inputNum "Number of inputs:"
      mask init:
      | bus_create_init(gcb,...
      |     'inputNum', inputNum);
  bus_expand1 : Subsystem  AncestorBlock=casper_library_flow_control/bus_expand  mask(bus_expand){mode=divisions of arbitrary size, outputNum=2, outputWidth=[1                                     32], outputBinaryPt=[0                                      0], outputArithmeticType=[2                                      0], show_format=on, outputToWorkspace=off, variablePrefix=adc0_d, outputToModelAsWell=on}
      mask prompts: outputNum "Number of outputs:"; outputWidth "Output width:"; outputBinaryPt "Output binary point position:"; outputArithmeticType "Output arithmetic type: (Unsigned=0, Signed=1, Boolean=2)"; show_format "Print format string?"; outputToWorkspace "Output to workspace?"; variablePrefix "Variable name prefix:"; outputToModelAsWell "Output to model as well?"
      mask help:
      | Expands a 'bus' made using a bus_create or Xilinx
      | concat block.
      | The input will be divided into the specified number
      | of outputs with the specified arithmetic types.
      | Divisions are made from most significant bit.
      mask init: same as c09f12_01_avn/bus_expand6
      settings: AttributesFormatString=2 outputs: b,uf32.0,
      mask TypeOptions mode: divisions of equal size | divisions of arbitrary size
      mask Callback mode: bus_expand_callback();
      mask Callback outputWidth: bus_expand_callback();
      mask Callback outputToWorkspace: bus_expand_callback();
  bus_expand3 : Subsystem  AncestorBlock=casper_library_flow_control/bus_expand  mask(bus_expand){mode=divisions of equal size, outputNum=4, outputWidth=8, outputBinaryPt=0, outputArithmeticType=0, show_format=on, outputToWorkspace=off, variablePrefix=adc0_d, outputToModelAsWell=on}
      mask prompts: outputNum "Number of outputs:"; outputWidth "Output width:"; outputBinaryPt "Output binary point position:"; outputArithmeticType "Output arithmetic type: (Unsigned=0, Signed=1, Boolean=2)"; show_format "Print format string?"; outputToWorkspace "Output to workspace?"; variablePrefix "Variable name prefix:"; outputToModelAsWell "Output to model as well?"
      mask help:
      | Expands a 'bus' made using a bus_create or Xilinx
      | concat block.
      | The input will be divided into the specified number
      | of outputs with the specified arithmetic types.
      | Divisions are made from most significant bit.
      mask init: same as c09f12_01_avn/bus_expand6
      settings: AttributesFormatString=4 outputs: uf8.0,uf8.0,uf8.0,uf8.0,
      mask TypeOptions mode: divisions of equal size | divisions of arbitrary size
      mask Callback mode: bus_expand_callback();
      mask Callback outputWidth: bus_expand_callback();
      mask Callback outputToWorkspace: bus_expand_callback();
  bus_expand4 : Subsystem  AncestorBlock=casper_library_flow_control/bus_expand  mask(bus_expand){mode=divisions of equal size, outputNum=4, outputWidth=8, outputBinaryPt=0, outputArithmeticType=0, show_format=on, outputToWorkspace=off, variablePrefix=adc0_d, outputToModelAsWell=on}
      mask prompts: outputNum "Number of outputs:"; outputWidth "Output width:"; outputBinaryPt "Output binary point position:"; outputArithmeticType "Output arithmetic type: (Unsigned=0, Signed=1, Boolean=2)"; show_format "Print format string?"; outputToWorkspace "Output to workspace?"; variablePrefix "Variable name prefix:"; outputToModelAsWell "Output to model as well?"
      mask help:
      | Expands a 'bus' made using a bus_create or Xilinx
      | concat block.
      | The input will be divided into the specified number
      | of outputs with the specified arithmetic types.
      | Divisions are made from most significant bit.
      mask init: same as c09f12_01_avn/bus_expand6
      settings: AttributesFormatString=4 outputs: uf8.0,uf8.0,uf8.0,uf8.0,
      mask TypeOptions mode: divisions of equal size | divisions of arbitrary size
      mask Callback mode: bus_expand_callback();
      mask Callback outputWidth: bus_expand_callback();
      mask Callback outputToWorkspace: bus_expand_callback();
  cd_tr : Subsystem  mask{cnt_bits=8, time_bits=48}
      mask prompts: cnt_bits "Bits in status counters"; time_bits "No LSBs in time to compare"
  cd_tr1 : Subsystem  mask{cnt_bits=8, time_bits=48}
      mask prompts: cnt_bits "Bits in status counters"; time_bits "No LSBs in time to compare"
  delay_coarse : Subsystem  AncestorBlock=casper_library/Delays/delay_wideband_prog  mask(delay_wideband_prog){max_delay=8192, n_inputs_bits=2, bram_latency=2, bram_type=Dual Port}
      mask prompts: max_delay "Max Delay (Sample Clks)"; n_inputs_bits "Number of Simultaneous Inputs(2^?)"; bram_latency "BRAM Latency"; bram_type "Select type of BRAM"
      mask init:
      | delay_wideband_prog_init(gcb,...
      |     'max_delay',max_delay,...
      |     'n_inputs_bits',n_inputs_bits,...
      |     'bram_latency',bram_latency,...
      |     'bram_type',bram_type);
      mask TypeOptions bram_type: Single Port | Dual Port
  delay_coarse1 : Subsystem  AncestorBlock=casper_library/Delays/delay_wideband_prog  mask(delay_wideband_prog){max_delay=8192, n_inputs_bits=2, bram_latency=2, bram_type=Dual Port}
      mask prompts: max_delay "Max Delay (Sample Clks)"; n_inputs_bits "Number of Simultaneous Inputs(2^?)"; bram_latency "BRAM Latency"; bram_type "Select type of BRAM"
      mask init:
      | delay_wideband_prog_init(gcb,...
      |     'max_delay',max_delay,...
      |     'n_inputs_bits',n_inputs_bits,...
      |     'bram_latency',bram_latency,...
      |     'bram_type',bram_type);
      mask TypeOptions bram_type: Single Port | Dual Port
  delay_gen0 : Subsystem  mask{fft_len=8, phase_bits=16, max_fringe_rate=23, min_fringe_rate=38, delay_bits=16+15, delay_bin_pt=16, max_delay_rate=23, min_delay_rate=38, add_latency=1, lookup_bits=11, cd_bits=13}
      mask prompts: fft_len "FFT size (2^?)"; phase_bits "Input phase resolution (2*pi/2^? radians)"; max_fringe_rate "Max fringe update rate (1/2^? radians/sample)"; min_fringe_rate "Min (non-zero) fringe rate (1/2^? radians/sample)"; delay_bits "Input delay resolution (bits)"; delay_bin_pt "Input delay binary point"; max_delay_rate "Max delay update rate (1/2^? samples/sample)"; min_delay_rate "Min (non-zero) delay update rate (1/2^? samples/sample)"; add_latency "Add latency"; lookup_bits "DDS lookup table resolution (2*pi/2^?)"; cd_bits "Coarse delay range (2^? bits)"
  delay_gen1 : Subsystem  mask{fft_len=8, phase_bits=16, max_fringe_rate=23, min_fringe_rate=38, delay_bits=16+15, delay_bin_pt=16, max_delay_rate=23, min_delay_rate=38, add_latency=1, lookup_bits=11, cd_bits=13}
      mask prompts: fft_len "FFT size (2^?)"; phase_bits "Input phase resolution (2*pi/2^? radians)"; max_fringe_rate "Max fringe update rate (1/2^? radians/sample)"; min_fringe_rate "Min (non-zero) fringe rate (1/2^? radians/sample)"; delay_bits "Input delay resolution (bits)"; delay_bin_pt "Input delay binary point"; max_delay_rate "Max delay update rate (1/2^? samples/sample)"; min_delay_rate "Min (non-zero) delay update rate (1/2^? samples/sample)"; add_latency "Add latency"; lookup_bits "DDS lookup table resolution (2*pi/2^?)"; cd_bits "Coarse delay range (2^? bits)"
  sync_out : Outport
  data4_0 : Outport  Port=2
  data4_1 : Outport  Port=3
  wires:
  cd_tr/1(arm_count) -> Terminator14/1
  mrst/1 -> cd_tr/1(rst), cd_tr1/1(rst)
  Logical12/1 -> cd_tr/3(arm)
  cd_lt/1 -> cd_tr/4(current_time), cd_tr1/4(current_time)
  arm0/1 -> Logical12/2
  cd_tr/2(ld_count) -> Terminator15/1
  cd_tr/3(value) -> Slice16/1, Slice19/1, Slice18/1, Slice15/1, Slice17/1
  cd_tr/4(enable) -> delay_gen0/2(en)
  ld_time0/1 -> cd_tr/5(load_time)
  ld_val0/1 -> cd_tr/6(load_value)
  load_now/1 -> Logical12/1, cd_tr/2(load_now), cd_tr1/2(load_now), Logical1/1
  delay_gen0/4(phase_out) -> Terminator1/1
  delay_gen0/5(slope_out) -> Terminator2/1
  delay_gen0/7(idx_d0) -> Terminator3/1
  delay_gen0/8(idx_d1) -> Terminator5/1
  Slice16/1 -> delay_gen0/3(phase)
  Slice19/1 -> delay_gen0/4(d/dt_phase)
  Slice18/1 -> Concat4/1
  Slice17/1 -> Concat4/2
  Concat4/1 -> delay_gen0/5(delay)
  Slice15/1 -> delay_gen0/6(d/dt_delay)
  Constant19/1 -> delay_gen0/8(invert_slope)
  delay_gen0/6(d0) -> bus_expand3/1(bus_in)
  delay_gen0/1(sync_out) -> delay_coarse/1(sync)
  delay_gen0/2(en_out) -> delay_coarse/3(en)
  delay_gen0/3(cd_o) -> delay_coarse/2(delay)
  delay_coarse/1(sync_out) -> sync_out/1
  delay_coarse/2(data_out1) -> bus_create4/1(in1)
  delay_coarse/3(data_out2) -> bus_create4/2(in2)
  delay_coarse/4(data_out3) -> bus_create4/3(in3)
  delay_coarse/5(data_out4) -> bus_create4/4(in4)
  bus_create4/1(bus_out) -> data4_0/1
  cd_tr/5(dout) -> bus_expand1/1(bus_in)
  bus_expand1/1(msb_out2) -> delay_gen0/1(sync_in), delay_gen1/1(sync_in)
  data0/1 -> bus_create1/2(in2)
  sync/1 -> bus_create1/1(in1)
  bus_create1/1(bus_out) -> cd_tr/7(din)
  cd_tr1/1(arm_count) -> Terminator6/1
  cd_tr1/2(ld_count) -> Terminator7/1
  cd_tr1/3(value) -> Slice3/1, Slice1/1, Slice4/1, Slice5/1, Slice2/1
  cd_tr1/4(enable) -> delay_gen1/2(en)
  delay_gen1/4(phase_out) -> Terminator4/1
  delay_gen1/5(slope_out) -> Terminator8/1
  delay_gen1/7(idx_d0) -> Terminator9/1
  delay_gen1/8(idx_d1) -> Terminator10/1
  Slice2/1 -> delay_gen1/3(phase)
  Slice5/1 -> delay_gen1/4(d/dt_phase)
  Slice4/1 -> Concat1/1
  Slice3/1 -> Concat1/2
  Concat1/1 -> delay_gen1/5(delay)
  Slice1/1 -> delay_gen1/6(d/dt_delay)
  Constant1/1 -> delay_gen1/8(invert_slope)
  delay_gen1/6(d0) -> bus_expand4/1(bus_in)
  delay_gen1/1(sync_out) -> delay_coarse1/1(sync)
  delay_gen1/2(en_out) -> delay_coarse1/3(en)
  delay_gen1/3(cd_o) -> delay_coarse1/2(delay)
  delay_coarse1/2(data_out1) -> bus_create2/1(in1)
  delay_coarse1/3(data_out2) -> bus_create2/2(in2)
  delay_coarse1/4(data_out3) -> bus_create2/3(in3)
  delay_coarse1/5(data_out4) -> bus_create2/4(in4)
  cd_tr1/5(dout) -> delay_gen1/7(din0)
  Logical1/1 -> cd_tr1/3(arm)
  arm1/1 -> Logical1/2
  ld_time1/1 -> cd_tr1/5(load_time)
  ld_val1/1 -> cd_tr1/6(load_value)
  data1/1 -> cd_tr1/7(din)
  bus_create2/1(bus_out) -> data4_1/1
  delay_coarse1/1(sync_out) -> Terminator11/1
  bus_expand4/1(msb_out4) -> delay_coarse1/4(data_in1)
  bus_expand4/2(out3) -> delay_coarse1/5(data_in2)
  bus_expand4/3(out2) -> delay_coarse1/6(data_in3)
  bus_expand4/4(lsb_out1) -> delay_coarse1/7(data_in4)
  bus_expand1/2(lsb_out1) -> delay_gen0/7(din0)
  bus_expand3/1(msb_out4) -> delay_coarse/4(data_in1)
  bus_expand3/2(out3) -> delay_coarse/5(data_in2)
  bus_expand3/3(out2) -> delay_coarse/6(data_in3)
  bus_expand3/4(lsb_out1) -> delay_coarse/7(data_in4)

== system c09f12_01_avn/convert ==
  note: 1000 -> 0
      | x100 -> 1
      | xx10 -> 2
      | xxx1 -> 3
  in : Inport
  Constant : xbsIndex_r4/Constant  const=0  gui_display_data_type=Fixed-point  arith_type=Unsigned  n_bits=2  bin_pt=0  preci_type=Single  exp_width=8  frac_width=24  explicit_period=off  period=1  equ=P=C  opselect=C  inp2=PCIN>>17  opr=+  inp1=P  carry=CIN  dbl_ovrd=off  block_type=constant
      settings: block_version=11.4
  Constant1 : xbsIndex_r4/Constant  const=0  gui_display_data_type=Fixed-point  arith_type=Unsigned  n_bits=2  bin_pt=0  preci_type=Single  exp_width=8  frac_width=24  explicit_period=off  period=1  equ=P=C  opselect=C  inp2=PCIN>>17  opr=+  inp1=P  carry=CIN  dbl_ovrd=off  block_type=constant
      settings: block_version=11.4
  Constant{8..15} (8 alike) : xbsIndex_r4/Constant  const=3  gui_display_data_type=Fixed-point  arith_type=Unsigned  n_bits=2  bin_pt=0  preci_type=Single  exp_width=8  frac_width=24  explicit_period=off  period=1  equ=P=C  opselect=C  inp2=PCIN>>17  opr=+  inp1=P  carry=CIN  dbl_ovrd=off  block_type=constant
      settings: block_version=11.4
  Constant2 : xbsIndex_r4/Constant  const=1  gui_display_data_type=Fixed-point  arith_type=Unsigned  n_bits=2  bin_pt=0  preci_type=Single  exp_width=8  frac_width=24  explicit_period=off  period=1  equ=P=C  opselect=C  inp2=PCIN>>17  opr=+  inp1=P  carry=CIN  dbl_ovrd=off  block_type=constant
      settings: block_version=11.4
  Constant3 : xbsIndex_r4/Constant  const=1  gui_display_data_type=Fixed-point  arith_type=Unsigned  n_bits=2  bin_pt=0  preci_type=Single  exp_width=8  frac_width=24  explicit_period=off  period=1  equ=P=C  opselect=C  inp2=PCIN>>17  opr=+  inp1=P  carry=CIN  dbl_ovrd=off  block_type=constant
      settings: block_version=11.4
  Constant{4..7} (4 alike) : xbsIndex_r4/Constant  const=2  gui_display_data_type=Fixed-point  arith_type=Unsigned  n_bits=2  bin_pt=0  preci_type=Single  exp_width=8  frac_width=24  explicit_period=off  period=1  equ=P=C  opselect=C  inp2=PCIN>>17  opr=+  inp1=P  carry=CIN  dbl_ovrd=off  block_type=constant
      settings: block_version=11.4
  Mux : xbsIndex_r4/Mux  inputs=16  en=off  latency=1  precision=Full  arith_type=Unsigned  n_bits=16  bin_pt=14  quantization=Truncate  overflow=Wrap  dbl_ovrd=off  block_type=mux
      settings: block_version=11.4
  Out1 : Outport
  wires:
  in/1 -> Mux/1
  Constant/1 -> Mux/2
  Constant1/1 -> Mux/3
  Constant2/1 -> Mux/4
  Constant3/1 -> Mux/5
  Constant4/1 -> Mux/6
  Constant5/1 -> Mux/7
  Constant6/1 -> Mux/8
  Constant7/1 -> Mux/9
  Constant8/1 -> Mux/10
  Constant9/1 -> Mux/11
  Constant10/1 -> Mux/12
  Constant12/1 -> Mux/13
  Constant13/1 -> Mux/14
  Constant11/1 -> Mux/15
  Constant15/1 -> Mux/16
  Constant14/1 -> Mux/17
  Mux/1 -> Out1/1

== system c09f12_01_avn/ct_tvg ==
  note: The TVG for the corner turner is just a ramp of fine channels, enabled by the data valid signal.
      | That's it. So after corner turning you'll just get the same value n times.
  syncin : Inport
  datain : Inport  Port=2
  validin : Inport  Port=3
  tvg_en : Inport  Port=4
  Convert : xbsIndex_r4/Convert  gui_display_data_type=Fixed-point  arith_type=Unsigned  n_bits=16  bin_pt=0  float_type=Single  exp_bits=8  fraction_bits=24  quantization=Truncate  overflow=Wrap  en=off  latency=0  dbl_ovrd=off  pipeline=off  block_type=convert
      settings: block_version=11.4
  Counter1 : xbsIndex_r4/Counter  cnt_type=Free Running  cnt_to=Inf  operation=Up  start_count=0  cnt_by_val=1  arith_type=Unsigned  n_bits=fine_bits  bin_pt=0  load_pin=off  rst=on  en=on  explicit_period=on  period=1  dbl_ovrd=off  use_behavioral_HDL=off  implementation=Fabric  block_type=counter
      settings: block_version=11.4
  Delay : xbsIndex_r4/Delay  rst=off  infoeditControl=Selection of Reset will increase slice count due to use of real FFs and instead of SRLs  en=off  latency=mux_latency  dbl_ovrd=off  reg_retiming=on  block_type=delay
      settings: block_version=11.4
  Delay1 : xbsIndex_r4/Delay  rst=off  infoeditControl=Selection of Reset will increase slice count due to use of real FFs and instead of SRLs  en=off  latency=mux_latency  dbl_ovrd=off  reg_retiming=on  block_type=delay
      settings: block_version=11.4
  Mux1 : xbsIndex_r4/Mux  inputs=2  en=off  latency=mux_latency  precision=Full  arith_type=Unsigned  n_bits=16  bin_pt=14  quantization=Truncate  overflow=Wrap  dbl_ovrd=off  block_type=mux
      settings: block_version=11.4
  scope : xbsIndex_r4/WaveScope  block_type=wavescope
      settings: block_version=11.4
  syncout : Outport
  dataout : Outport  Port=2
  validout : Outport  Port=3
  wires:
  syncin/1 -> Counter1/1, Delay/1  "syncin"
  validin/1 -> Counter1/2, Delay1/1  "validin"
  datain/1 -> Mux1/2  "datain"
  tvg_en/1 -> Mux1/1  "tvg_en"
  Counter1/1 -> Convert/1  "tvgdata"
  Mux1/1 -> dataout/1
  Delay/1 -> syncout/1
  Delay1/1 -> validout/1
  Convert/1 -> Mux1/3
